simulink model "aeropendulum_model"  (Simulink 9.0)
settings: Solver=VariableStepAuto  StartTime=0.0  StopTime=10.0  RelTol=1e-3
values from neighbouring files (symbols this model uses):
  c = 0.01    [Main.m]
  d = 0.023    [Main.m]
  g = 9.80665    [Main.m]
  J = 0.0090    (= 0.009)    [Main.m]
  L = 0.495    [Main.m]
  m = 0.43    [Main.m]
libraries: simulink_extras x1
settings Model: Creator=emerrf  LastModifiedBy=emerrf
settings DataIOCC: SaveFormat=Dataset
settings OptimizationCC: LifeSpan=auto
settings DebuggingCC: UnderspecifiedInitializationDetection=Simplified  MergeDetectMultiDrivingBlocksExec=error  SFUnexpectedBacktrackingDiag=error  SFNoUnconditionalDefaultTransitionDiag=error  SFExecutionAtInitializationDiag=warning
settings HardwareCC: ProdBitPerPointer=64  ProdBitPerSizeT=64  ProdBitPerPtrDiffT=64  ProdLargestAtomicFloat=Float  ProdIntDivRoundTo=Zero  ProdEndianess=LittleEndian  ProdWordSize=64  ProdHWDeviceType=Intel->x86-64 (Windows64)
settings ModelReferenceCC: PropagateSignalLabelsOutOfModel=on
settings CodeAppCC: StateflowObjectComments=off
settings GRTTargetCC: TargetLangStandard=C99 (ISO)
settings ConfigComp: CovMetricSettings=dwe  CovHtmlReporting=off  CovSaveCumulativeToWorkspaceVar=off  CovSaveSingleToWorkspaceVar=off  CovExternalEMLEnable=on

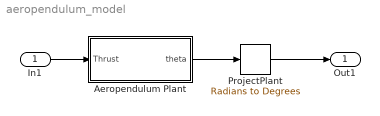
== system aeropendulum_model ==
  In1 : Inport
  Aeropendulum Plant : Subsystem
  ProjectPlant : simulink_extras/Transformations/Radians to Degrees
  Out1 : Outport
  wires:
  Aeropendulum Plant/1(theta) -> ProjectPlant/1
  In1/1 -> Aeropendulum Plant/1(Thrust)
  ProjectPlant/1 -> Out1/1

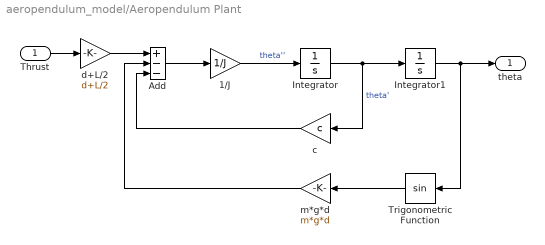
== system aeropendulum_model/Aeropendulum Plant ==
  Thrust : Inport
  1/J : Gain  Gain=1/J
  Add : Sum  Inputs=+--
  Integrator : Integrator
  Integrator1 : Integrator
  Trigonometric Function : Trigonometry
  c : Gain  Gain=c
  d+L/2 : Gain  Gain=d+L/2
  m*g*d : Gain  Gain=m*g*d
  theta : Outport
  wires:
  Thrust/1 -> d+L/2/1
  Add/1 -> 1/J/1
  1/J/1 -> Integrator/1  "theta''"
  Integrator/1 -> c/1, Integrator1/1  "theta'"
  Integrator1/1 -> Trigonometric Function/1, theta/1
  Trigonometric Function/1 -> m*g*d/1
  m*g*d/1 -> Add/2
  c/1 -> Add/3
  d+L/2/1 -> Add/1
